simulink model "PID"  (R2021b)
settings: Solver=VariableStepAuto  StartTime=0.0  StopTime=20  RelTol=1e-3
libraries: slpidlib x1
settings Model: Creator=rafae  LastModifiedBy=rafae

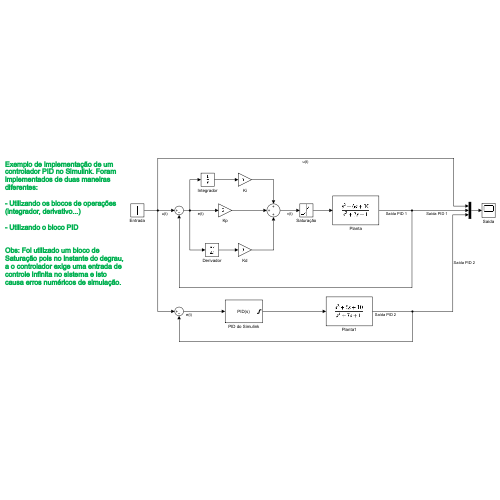
[thumbnail: Simulink's stored preview of the top-level diagram]
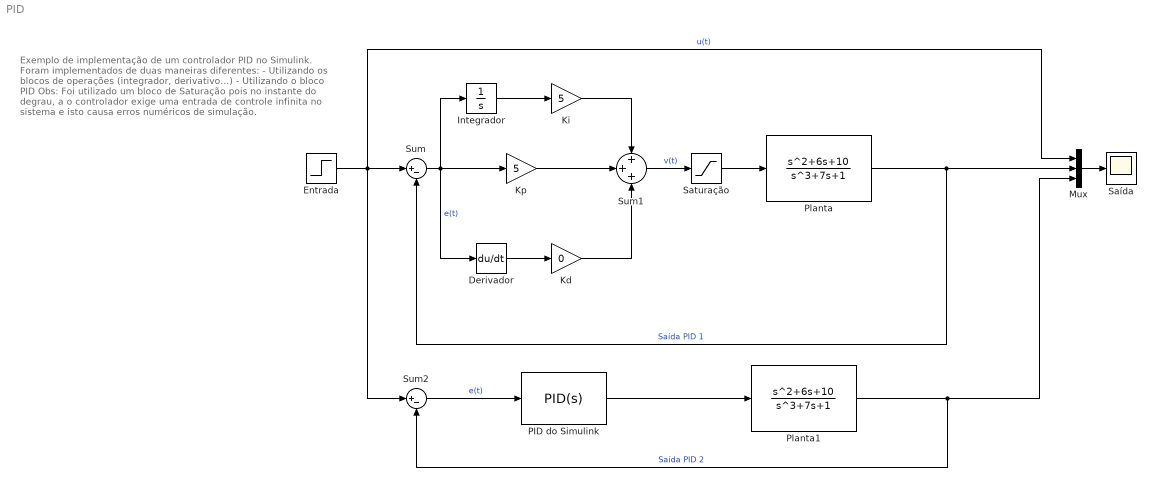
== system PID ==
  note: Exemplo de implementação de um controlador PID no Simulink. Foram implementados de duas maneiras diferentes:
      |
      | - Utilizando os blocos de operações (integrador, derivativo...)
      |
      | - Utilizando o bloco PID
      |
      | Obs: Foi utilizado um bloco de Saturação pois no instante do degrau, a o controlador exige uma entrada de controle infinita no sistema e isto causa erros numéricos de simulação.
  Derivador : Derivative
  Entrada : Step  SampleTime=0
  Integrador : Integrator
  Kd : Gain  Gain=0
  Ki : Gain  Gain=5
  Kp : Gain  Gain=5
  Mux : Mux  Inputs=3
  PID do Simulink : slpidlib/PID Controller  Controller=PID  Form=Parallel  TimeDomain=Continuous-time  UseExternalTs=off  SampleTime=-1  IntegratorMethod=Forward Euler  FilterMethod=Forward Euler  ControllerParametersSource=internal  P=5  I=5  D=0  UseFilter=on  N=100  TunerSelectOption=Transfer Function Based (PID Tuner App)  InitialConditionSource=internal  InitialConditionForIntegrator=0  InitialConditionForFilter=0  DifferentiatorICPrevScaledInput=0  ExternalReset=none  TrackingMode=off  Kt=1  LimitOutput=on  SatLimitsSource=internal  UpperSaturationLimit=2  LowerSaturationLimit=-2  LinearizeAsGain=on  AntiWindupMode=none  Kb=1  POutMin=[]  POutMax=[]  IOutMin=[]  IOutMax=[]  DOutMin=[]  DOutMax=[]  NOutMin=[]  NOutMax=[]  SumOutMin=[]  SumOutMax=[]  SaturationOutMin=[]  SaturationOutMax=[]  PParamMin=[]  PParamMax=[]  IParamMin=[]  IParamMax=[]  DParamMin=[]  DParamMax=[]  NParamMin=[]  NParamMax=[]  KbParamMin=[]  KbParamMax=[]  KtParamMin=[]  KtParamMax=[]  KbOutMin=[]  KbOutMax=[]  KtOutMin=[]  KtOutMax=[]  IntegratorOutMin=[]  IntegratorOutMax=[]  FilterOutMin=[]  FilterOutMax=[]  SumI1OutMin=[]  SumI1OutMax=[]  SumI2OutMin=[]  SumI2OutMax=[]  SumI3OutMin=[]  SumI3OutMax=[]  SumI4OutMin=[]  SumI4OutMax=[]  SumDOutMin=[]  SumDOutMax=[]  DifferentiatorOutMin=[]  DifferentiatorOutMax=[]  FilterDiffOutCoefMin=[]  FilterDiffOutCoefMax=[]  ReciprocalOutMin=[]  ReciprocalOutMax=[]  SumDenOutMin=[]  SumDenOutMax=[]  SumNumOutMin=[]  SumNumOutMax=[]  DivideOutMin=[]  DivideOutMax=[]  UdiffTsProdOutMin=[]  UdiffTsProdOutMax=[]  NTsProdOutMin=[]  NTsProdOutMax=[]  UintegralTsProdOutMin=[]  UintegralTsProdOutMax=[]  UngainTsProdOutMin=[]  UngainTsProdOutMax=[]  IntegratorContinuousStateAttributes=''  IntegratorStateMustResolveToSignalObject=off  IntegratorRTWStateStorageClass=Auto  FilterContinuousStateAttributes=''  FilterStateMustResolveToSignalObject=off  FilterRTWStateStorageClass=Auto  ParallelPVariant=InternalParameters  IdealPVariant=Disabled  IVariant=InternalParameters  DVariant=InternalParameters  IntegratorVariant=Continuous  SatVariant=Enabled  AWVariant=Passthrough  PCopyVariant=Disabled  TRVariant=Disabled  FdbkBlocksVariant=Forward  IdealPFdbkVariant=Disabled  SatFdbkVariant=Disabled  DerivativeFilterVariant=ContFilter  NVariant=InternalParameters  NCopyVariant=Disabled  FilterICVariant=InternalICsFilter  IntegratorICVariant=InternalICs  ExternalResetVariant=Disabled  TRSumVariant=Passthrough  SumFdbkVariant=Disabled  SumVariant=Sum_PID  TsampFilterVariant=InternalTs  TsampNgainVariant=Passthrough  TsampIntegralVariant=Passthrough  ExternalSaturationOutDataTypeStr=Inherit: Same as second input
  Planta : TransferFcn  Numerator=[1,6,10]  Denominator=[1,0,7,1]
  Planta1 : TransferFcn  Numerator=[1,6,10]  Denominator=[1,0,7,1]
  Saturação : Saturate  UpperLimit=2  LowerLimit=-2
  Saída : Scope
  Sum : Sum  Inputs=|+-
  Sum1 : Sum  Inputs=+++
  Sum2 : Sum  Inputs=|+-
  wires:
  Entrada/1 -> Sum2/1, Mux/1, Sum/1  "u(t)"
  Planta/1 -> Mux/2, Sum/2  "Saída PID 1"
  Sum/1 -> Derivador/1, Integrador/1, Kp/1  "e(t)"
  Kp/1 -> Sum1/2
  Mux/1 -> Saída/1
  Integrador/1 -> Ki/1
  Sum1/1 -> Saturação/1  "v(t)"
  Ki/1 -> Sum1/1
  Derivador/1 -> Kd/1
  Kd/1 -> Sum1/3
  Saturação/1 -> Planta/1
  PID do Simulink/1 -> Planta1/1
  Sum2/1 -> PID do Simulink/1  "e(t)"
  Planta1/1 -> Mux/3, Sum2/2  "Saída PID 2"
